simulink model "SHEV_Camaro_PwrLossMdl"  (R2018b)
settings: Solver=ode2  StartTime=0.0  StopTime=simDrv.time_s(end)  FixedStep=t_step  RelTol=1e-3
values from neighbouring files (symbols this model uses):
  A123_ESS =     [PwrLossMdl_A123Battery.mat]
  adj_motEffMap = [0.25 0.31 0.37 0.38 0.4 0.49 0.58 0.64 0.31 0.36 0.39 0.406 ... (72 elements, 8x9)]    [PwrLossMdl_PropSysEffData.mat]
  adjbsfc_map = [1051 1388 1174 1085 895 602 501 388 388 1051 1134 996 ... (81 elements, 9x9)]    [PwrLossMdl_GenSysEffData.mat]
  adjbsfc_spdbpt = [4003 4510 4987 5412 5800 5986 6322 6643 6889]    [PwrLossMdl_GenSysEffData.mat]
  adjbsfc_trqbpt = [10 15 20 25 30 35 40 45 50]    [PwrLossMdl_GenSysEffData.mat]
  C1 = [20000 20000 46318.5184323 46009.1793978 1021.23087801 1108.29786665 9922.48088723 10264.7269718 18293.5148586 29962.1621632 36298.3673472 37544.2700719 ... (41 elements, 1x41)]    [PwrLossMdl_ESS.mat]
  C2 = [20000 20000 46318.5184106 46009.1793608 1021.23035996 1108.29602087 9922.4809203 10264.72697 18293.5148606 29962.1621637 36298.3673482 37544.2700716 ... (41 elements, 1x41)]    [PwrLossMdl_ESS.mat]
  contMotTrq = [250 250 250 250 250 250 225 190 170]    [PwrLossMdl_PropSysEffData.mat]    (also in startPwrLossMdl.m = [180;180;180;180;180;180;180;180;170])
  cs_ll = 0.15    [startPwrLossMdl.m]
  cs_ul = 0.25    [startPwrLossMdl.m]
  E85_LHV = 30000    [startPwrLossMdl.m]
  mot_gbx_rat = 4.2    [startPwrLossMdl.m]
  motSpdVec = [1 500 1000 1500 2000 2500 3000 3500 4000]    [PwrLossMdl_PropSysEffData.mat]
  motTrqVec = [1 25 50 75 100 125 150 175]    [PwrLossMdl_PropSysEffData.mat]
  R0 = [0.5 0.5 0.413858741447 0.181330616185 0.123924684061 0.082623865753 0.114591066521 0.096554690516 0.0949331545326 0.124564294889 0.118490098825 0.107959033825 ... (41 elements, 1x41)]    [PwrLossMdl_ESS.mat]
  R1 = [0.5 0.5 0.513602817558 0.526624804767 0.484906164492 0.489343525408 0.493637128787 0.498122066152 0.500091294983 0.500054252951 0.500314275839 0.500483147312 ... (41 elements, 1x41)]    [PwrLossMdl_ESS.mat]
  R2 = [0.5 0.5 0.513602817535 0.526624804695 0.484906164494 0.489343525401 0.493637128787 0.498122066152 0.500091294984 0.50005425295 0.500314275838 0.500483147311 ... (41 elements, 1x41)]    [PwrLossMdl_ESS.mat]
  rho_fuel_gpL = 783    [startPwrLossMdl.m]
  simDrv = EEC_Single    [startPwrLossMdl.m]
  soc_bpt = [0 0.025 0.05 0.075 0.1 0.125 0.15 0.175 0.2 0.225 0.25 0.275 ... (41 elements, 1x41)]    [PwrLossMdl_ESS.mat]
  t_step = 0.1    [startPwrLossMdl.m]
  tire_rad_m = 0.346    [startPwrLossMdl.m]
  V_fuel_init_gal = 7    [startPwrLossMdl.m]
undefined symbols (not defined in the file or in its folder): DiscIntNeverNeededParam, N_OptResults, OptResults
libraries: simulink x10, custom_func x2, dspstat3 x1
(part 1 of 2)
PauseFcn:
  | runOptSHEV_DP_FwdProp
settings Model: Creator=Aman-Home  LastModifiedBy=Aman-Home

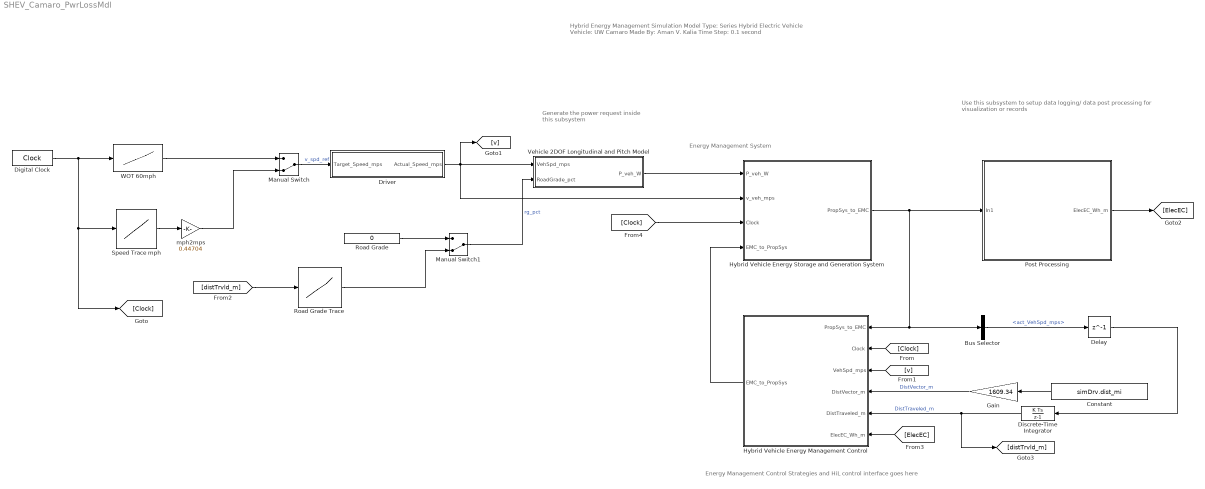
== system SHEV_Camaro_PwrLossMdl ==
  note: Energy Management Control Strategies and HiL control interface goes here
  note: Hybrid Energy Management Simulation Model
      | Type: Series Hybrid Electric Vehicle
      | Vehicle: UW Camaro
      | Made By: Aman V. Kalia
      | Time Step: 0.1 second
  note: Use this subsystem to setup data logging/ data post processing
      | for visualization or records
  note: Generate the power request inside
      | this subsystem
  note: Energy Management System
  Bus Selector : BusSelector  OutputSignals=act_VehSpd_mps
  Constant : Constant  Value=simDrv.dist_mi
  Delay : Delay  DelayLength=1
  Digital Clock : DigitalClock  SampleTime=t_step
  Discrete-Time Integrator : DiscreteIntegrator  SampleTime=t_step  ICPrevOutput=DiscIntNeverNeededParam  ICPrevScaledInput=DiscIntNeverNeededParam
  Driver : Subsystem
  Gain : Gain  Gain=1609.34
  Hybrid Vehicle Energy Management Control : Subsystem
  Hybrid Vehicle Energy Storage and Generation System : Subsystem
  Manual Switch : ManualSwitch  CurrentSetting=0
  Manual Switch1 : ManualSwitch  CurrentSetting=0
  Post Processing : Subsystem
  Road Grade : Constant  Value=0
  Road Grade Trace : Lookup_n-D  NumberOfTableDimensions=1  BreakpointsForDimension1=simDrv.dist_mi(1:end-1) * 1609.34  Table=simDrv.grade_pct(1:end-1)  ExtrapMethod=Clip  UseLastTableValue=on  InternalRulePriority=Speed  RndMeth=Simplest  InputSameDT=on
  Speed Trace mph : Lookup_n-D  NumberOfTableDimensions=1  BreakpointsForDimension1=simDrv.time_s  Table=simDrv.rand_spd_mph  ExtrapMethod=Clip  InternalRulePriority=Speed  RndMeth=Simplest  InputSameDT=on
  Vehicle 2DOF Longitudinal and Pitch Model : Subsystem
  WOT 60mph : Lookup_n-D  NumberOfTableDimensions=1  BreakpointsForDimension1=[0,5,10,simDrv.time_s(end)]  Table=[0,0,60,60] * 0.447  ExtrapMethod=Clip  InternalRulePriority=Speed  RndMeth=Simplest  InputSameDT=on
  mph2mps : Gain  Gain=0.44704
  wires:
  Manual Switch/1 -> Driver/1(Target_Speed_mps)  "v_spd_ref"
  Hybrid Vehicle Energy Management Control/1(EMC_to_PropSys) -> Hybrid Vehicle Energy Storage and Generation System/4(EMC_to_PropSys)
  Hybrid Vehicle Energy Storage and Generation System/1(PropSys_to_EMC) -> Hybrid Vehicle Energy Management Control/1(PropSys_to_EMC), Bus Selector/1, Post Processing/1(In1)
  Vehicle 2DOF Longitudinal and Pitch Model/1(P_veh_W) -> Hybrid Vehicle Energy Storage and Generation System/1(P_veh_W)
  Manual Switch1/1 -> Vehicle 2DOF Longitudinal and Pitch Model/2(RoadGrade_pct)  "rg_pct"
  Digital Clock/1 -> [Clock], Speed Trace mph/1, WOT 60mph/1
  Speed Trace mph/1 -> mph2mps/1
  Road Grade/1 -> Manual Switch1/1
  Road Grade Trace/1 -> Manual Switch1/2
  [Clock] -> Hybrid Vehicle Energy Management Control/2(Clock)
  [v] -> Hybrid Vehicle Energy Management Control/3(VehSpd_mps)
  Constant/1 -> Gain/1
  Bus Selector/1 -> Delay/1  "<act_VehSpd_mps>"
  Discrete-Time Integrator/1 -> [distTrvld_m], Hybrid Vehicle Energy Management Control/5(DistTraveled_m)  "DistTraveled_m"
  Gain/1 -> Hybrid Vehicle Energy Management Control/4(DistVector_m)  "DistVector_m"
  WOT 60mph/1 -> Manual Switch/1
  Post Processing/1(ElecEC_Wh_m) -> [ElecEC]
  [ElecEC] -> Hybrid Vehicle Energy Management Control/6(ElecEC_Wh_m)
  Driver/1(Actual_Speed_mps) -> Hybrid Vehicle Energy Storage and Generation System/2(v_veh_mps), Vehicle 2DOF Longitudinal and Pitch Model/1(VehSpd_mps), [v]
  [Clock] -> Hybrid Vehicle Energy Storage and Generation System/3(Clock)
  mph2mps/1 -> Manual Switch/2
  Delay/1 -> Discrete-Time Integrator/1
  [distTrvld_m] -> Road Grade Trace/1

== system SHEV_Camaro_PwrLossMdl/Driver ==
  Target_Speed_mps : Inport
  Actual_Speed_mps : Outport
  wires:
  Target_Speed_mps/1 -> Actual_Speed_mps/1

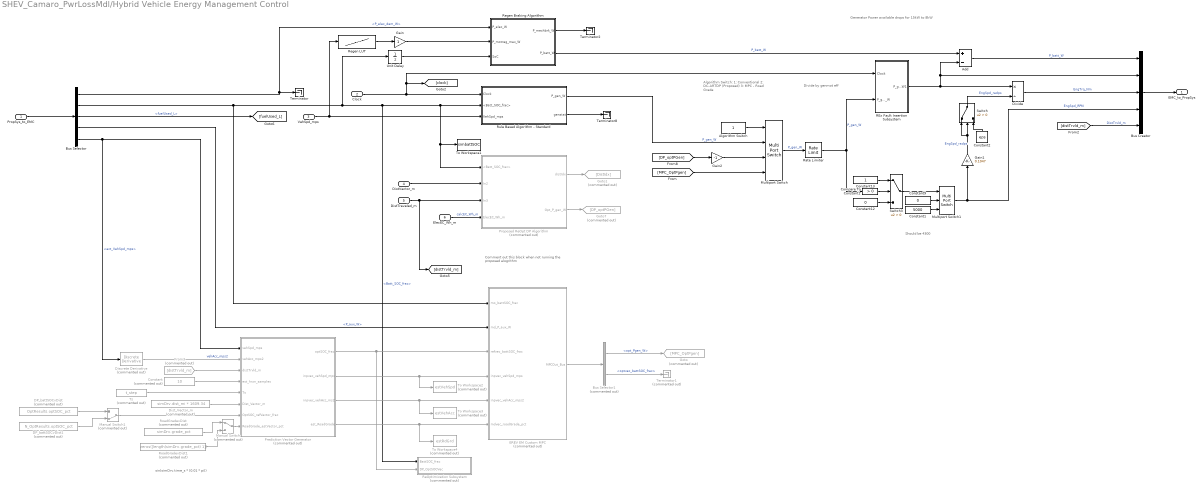
== system SHEV_Camaro_PwrLossMdl/Hybrid Vehicle Energy Management Control ==
  note: Divide by genmot eff
  note: Should be 4300
  note: sin(simDrv.time_s * (0.01 * pi))
  note: Algorithm Switch:
      | 1: Conventional
      | 2: DC-ARTDP (Proposed)
      | 3: MPC - Road Grade
  note: Comment out this block when not
      | running the proposed alogrithm
  note: Generator Power available drops for 15kW to 8kW
  PropSys_to_EMC : Inport
  Clock : Inport  Port=2
  VehSpd_mps : Inport  Port=3
  DistVector_m : Inport  Port=4
  DistTraveled_m : Inport  Port=5
  ElecEC_Wh_m : Inport  Port=6
  Add : Sum  Inputs=+-
  Algorithm Switch : Constant
  Bus Creator : BusCreator  Inputs=5
  Bus Selector : BusSelector  OutputSignals=P_elec_dem_W,Batt_SOC_frac,fuelUsed_L,P_aux_W,act_VehSpd_mps
  Bus Selector1 : BusSelector  Commented=on  OutputSignals=opt_Pgen_W,optvec_battSOC_frac
  Compare To Constant1 : simulink/Logic and Bit Operations/Compare To Constant  relop=>  const=0  OutDataTypeStr=boolean
  Constant : Constant  Commented=on  Value=10
  Constant1 : Constant  Value=5000
  Constant12 : Constant  Value=0
  Constant13 : Constant
  Constant2 : Constant  Value=eps
  Constant9 : Constant  Value=0
  DP_battSOCvDist : Constant  Commented=on  Value=OptResults.optSOC_pct
  DP_battSOCvDist1 : Constant  Commented=on  Value=N_OptResults.optSOC_pct
  Discrete Derivative : simulink/Discrete/Discrete Derivative  Commented=on  gainval=1.0  ICPrevScaledInput=0.0  OutMin=[]  OutMax=[]  OutDataType=fixdt(1, 16)  OutScaling=2^-10  DoSatur=off
  Dist_Vector_m : Constant  Commented=on  Value=simDrv.dist_mi * 1609.34
  Divide : Product  Inputs=*/
  EREV EM Custom MPC : Subsystem  Commented=on  mask{msk_init_Pgen=0, msk_est_hrzn_samples=10, msk_ctl_hrzn_samples=10, msk_t_step=1}
      mask prompts: msk_init_Pgen "Initial generator power [W]:"; msk_est_hrzn_samples "Estimation horizon samples [-]:"; msk_ctl_hrzn_samples "Control horizon samples [-]:"; msk_t_step "Time step [-]:"
      mask DialogControl DescGroupVar Prompt: Custom EREV MPC
      mask DialogControl DescTextVar Prompt: This block implements a custom MPC Energy Management algorithm for the EREV Camaro.
      mask DialogControl ParameterGroupVar Prompt: MPC Parameters
  From3 : From  Commented=on  GotoTag=distTrvld_m
  Gain : Gain
  Gain1 : Gain  Gain=0.1047
  Gain2 : Gain  Gain=-1
  Goto : Goto  Commented=on  GotoTag=MPC_OptPgen
  Goto1 : Goto  Commented=on  GotoTag=DistIdx
  Goto7 : Goto  Commented=on  GotoTag=DP_optPGen
  Manual Switch : ManualSwitch  Commented=on
  Manual Switch1 : ManualSwitch  Commented=on  CurrentSetting=0
  Multiport Switch : MultiPortSwitch
  Multiport Switch1 : MultiPortSwitch  DataPortOrder=Zero-based contiguous  Inputs=2  zeroidx=on
  Prediction Vector Generator : Subsystem  Commented=on
  Proposed ReOpt DP Algorithm : Subsystem  Commented=on
  REx Fault Insertion Subsystem : Subsystem  mask{FaultTypes=No Fault, t_shutfault=6000}
      mask prompts: FaultTypes "Select Fault Type:"; t_shutfault "Enter the time marker [s]:"
      mask init:
      | switch FaultTypes
      |     case 'No Fault'
      |         FaultDec = 0;
      |         %set_param('SHEV_Camaro_PwrLossMdl/Hybrid Vehicle Energy Management Control/Fault Insertion Subsystem','choice','0')
      |     case 'Deration Fault'
      |         FaultDec = 1;
      |         %set_param('SHEV_Camaro_PwrLossMdl/Hybrid Vehicle Energy Management Control/REx Fault Insertion Subsystem','choice','1')
      |     case 'Shut Down Fault'
      |         FaultDec = 2;
      |         %set_param('SHEV_Camaro_PwrLossMdl/Hybrid Vehicle Energy Management Control/Fault Insertion Subsystem','choice','2')
      | end
      mask TypeOptions FaultTypes: No Fault | Deration Fault | Shut Down Fault
      mask Callback FaultTypes:
      | % Get the mask parameter values. This is a cell
      | %   array of character vectors.
      | maskStr = get_param(gcb,'FaultTypes');
      | 
      | % The pop-up menu is the first mask parameter.
      | %   Check the value selected in the pop-up
      | if strcmp(maskStr(1),'S'),
      | 
      |     % Set the visibility of both parameters on when
      |     %   User-defined is selected in the pop-up.
      | 
      |     set_param(gcb,'MaskVisibilities',{'on';'on'}),
      | 
      | else
      | 
      |     % Turn off the visibility of the Value field
      |     %   when User-defined is not selected.
      | 
      |     set_param(gcb,'MaskVisibilities',{'on';'off'}),
      | 
      |     % Set the character vector in the Values field equal to the
      |     % character vector selected in the Gain pop-up menu.
      | 
      |     %maskStr{2}=maskStr{1};
      |     %set_param(gcb,'t_shutfault',inf);
      | end
      mask DialogControl DescGroupVar Prompt: Fault Insertion Block
      mask DialogControl DescTextVar Prompt: Select "Insert Fault" to enable fault insertion. Deselect to turn it off.
      mask DialogControl DescVar Prompt: Select the fault level [0,1,2] using the dial below. [0: No Fault, 1: Deration Fault, 2: Shut Off]
  Rate Limiter : RateLimiter  RisingSlewLimit=250  FallingSlewLimit=-4500  SampleTimeMode=inherited
  ReOptimization Subsystem : Subsystem  Commented=on
  Regen Braking Algorithm : Stateflow chart  TreatAsAtomicUnit=on
  Regen LUT : Lookup_n-D  NumberOfTableDimensions=1  BreakpointsForDimension1=[0 2.6 5.2 7.8 10.4 13 15.6 18.2 20.8 23.4 26 28.6 31.2 33.8 38]  Table=[0 0 -1250 -3000 -5500 -8000 -10250 -12500 -13750 -14000 -14500 -15000 -15000 -15000 -15000]  InternalRulePriority=Speed  RndMeth=Simplest  InputSameDT=on
  RoadGradevDist : Constant  Commented=on  Value=simDrv.grade_pct
  RoadGradevDist1 : Constant  Commented=on  Value=zeros([length(simDrv.grade_pct) 1])
  Rule Based Algorithm - Standard : Subsystem
  Switch : Switch  Criteria=u2 > Threshold
  Switch3 : Switch  Criteria=u2 > Threshold
  Terminator : Terminator
  Terminator1 : Terminator  Commented=on
  Terminator2 : Terminator
  Terminator8 : Terminator
  To Workspace1 : ToWorkspace  VariableName=simbattSOC  SaveFormat=Timeseries  SampleTime=1
  To Workspace2 : ToWorkspace  Commented=on  VariableName=estVehSpd  SaveFormat=Structure With Time  SampleTime=-1
      settings: Save2DSignal=2-D array (concatenate along first dimension)
  To Workspace3 : ToWorkspace  Commented=on  VariableName=estVehAcc  SaveFormat=Structure With Time  SampleTime=-1
      settings: Save2DSignal=2-D array (concatenate along first dimension)
  To Workspace4 : ToWorkspace  Commented=on  VariableName=estRdGrd  SaveFormat=Structure With Time  SampleTime=-1
      settings: Save2DSignal=2-D array (concatenate along first dimension)
  Ts : Constant  Commented=on  Value=t_step
  Unit Delay : UnitDelay  SampleTime=-1
  EMC_to_PropSys : Outport
  wires:
  Bus Creator/1 -> EMC_to_PropSys/1
  Add/1 -> Bus Creator/1  "P_batt_W"
  Divide/1 -> Bus Creator/3  "EngTrq_Nm"
  Multiport Switch1/1 -> Gain1/1, Bus Creator/4  "EngSpd_RPM"
  PropSys_to_EMC/1 -> Bus Selector/1
  Bus Selector/1 -> Terminator/1, Regen Braking Algorithm/1(P_elec_W)  "<P_elec_dem_W>"
  Regen LUT/1 -> Gain/1
  Regen Braking Algorithm/1(P_mechbrk_W) -> Terminator2/1
  Gain/1 -> Regen Braking Algorithm/2(P_motreg_max_W)
  Constant9/1 -> Multiport Switch1/2
  Constant1/1 -> Multiport Switch1/3
  Switch/1 -> Divide/2  "EngSpd_radps"
  Gain1/1 -> Switch/1, Switch/2  "EngSpd_radps"
  Constant2/1 -> Switch/3
  Regen Braking Algorithm/2(P_batt_W) -> Add/1  "P_batt_W"
  Clock/1 -> Rule Based Algorithm - Standard/1(Clock), REx Fault Insertion Subsystem/1(Clock), [clock]
  Bus Selector/2 -> EREV EM Custom MPC/1(mo_battSOC_frac), ReOptimization Subsystem/1(BattSOC_frac), Rule Based Algorithm - Standard/2(<Batt_SOC_frac>), Proposed ReOpt DP Algorithm/1(<Batt_SOC_frac>), To Workspace1/1, Unit Delay/1  "<Batt_SOC_frac>"
  VehSpd_mps/1 -> Rule Based Algorithm - Standard/3(VehSpd_mps), Regen LUT/1
  Switch3/1 -> Multiport Switch1/1
  DistTraveled_m/1 -> Proposed ReOpt DP Algorithm/3(In3), [distTrvld_m]
  Bus Selector/3 -> [fuelUsed_L]  "<fuelUsed_L>"
  [DP_optPGen] -> Gain2/1
  Gain2/1 -> Multiport Switch/3
  Rule Based Algorithm - Standard/1(P_gen_W) -> Multiport Switch/2  "P_gen_W"
  Algorithm Switch/1 -> Multiport Switch/1
  Rule Based Algorithm - Standard/2(genstat) -> Terminator8/1
  Compare To Constant1/1 -> Switch3/2
  Constant12/1 -> Switch3/3
  Constant13/1 -> Switch3/1
  [distTrvld_m] -> Bus Creator/5  "DistTrvld_m"
  Unit Delay/1 -> Regen Braking Algorithm/3(SoC)
  REx Fault Insertion Subsystem/1(P_gen_W1) -> Add/2, Bus Creator/2, Divide/1
  Rate Limiter/1 -> Compare To Constant1/1, REx Fault Insertion Subsystem/2(P_gen_W)  "P_gen_W"
  DistVector_m/1 -> Proposed ReOpt DP Algorithm/2(In2)
  ElecEC_Wh_m/1 -> Proposed ReOpt DP Algorithm/4(ElecEC_Wh_m)  "calcEC_Wh_m"
  Proposed ReOpt DP Algorithm/1(distIdx) -> Goto1/1
  Proposed ReOpt DP Algorithm/2(Opt_P_gen_W) -> Goto7/1
  [MPC_OptPgen] -> Multiport Switch/4
  EREV EM Custom MPC/1(MPCOut_Bus) -> Bus Selector1/1
  Bus Selector1/1 -> Goto/1  "<opt_Pgen_W>"
  Bus Selector1/2 -> Terminator1/1  "<optvec_battSOC_frac>"
  Bus Selector/4 -> EREV EM Custom MPC/2(md_P_aux_W)  "<P_aux_W>"
  Prediction Vector Generator/1(optSOC_frac) -> ReOptimization Subsystem/2(DP_OptSOCVec), EREV EM Custom MPC/3(refvec_battSOC_frac)
  Prediction Vector Generator/2(inpvec_vehSpd_mps) -> To Workspace2/1, EREV EM Custom MPC/4(inpvec_vehSpd_mps)
  Prediction Vector Generator/3(inpvec_vehAcc_ms2) -> To Workspace3/1, EREV EM Custom MPC/5(inpvec_vehAcc_mps2)
  Prediction Vector Generator/4(est_RoadGrade) -> To Workspace4/1, EREV EM Custom MPC/6(mdvec_roadGrade_pct)
  From3/1 -> Prediction Vector Generator/3(distTrvld_m)
  Constant/1 -> Prediction Vector Generator/4(est_hrzn_samples)
  RoadGradevDist/1 -> Manual Switch/1
  Manual Switch1/1 -> Prediction Vector Generator/7(OptSOC_refVector_frac)
  Dist_Vector_m/1 -> Prediction Vector Generator/6(Dist_Vector_m)
  Ts/1 -> Prediction Vector Generator/5(Ts)
  Bus Selector/5 -> Discrete Derivative/1, Prediction Vector Generator/1(vehSpd_mps)  "<act_VehSpd_mps>"
  Discrete Derivative/1 -> Prediction Vector Generator/2(vehAcc_mps2)  "vehAcc_mps2"
  Manual Switch/1 -> Prediction Vector Generator/8(RoadGrade_estVector_pct)
  RoadGradevDist1/1 -> Manual Switch/2
  DP_battSOCvDist/1 -> Manual Switch1/1
  DP_battSOCvDist1/1 -> Manual Switch1/2
  Multiport Switch/1 -> Rate Limiter/1  "P_gen_W"

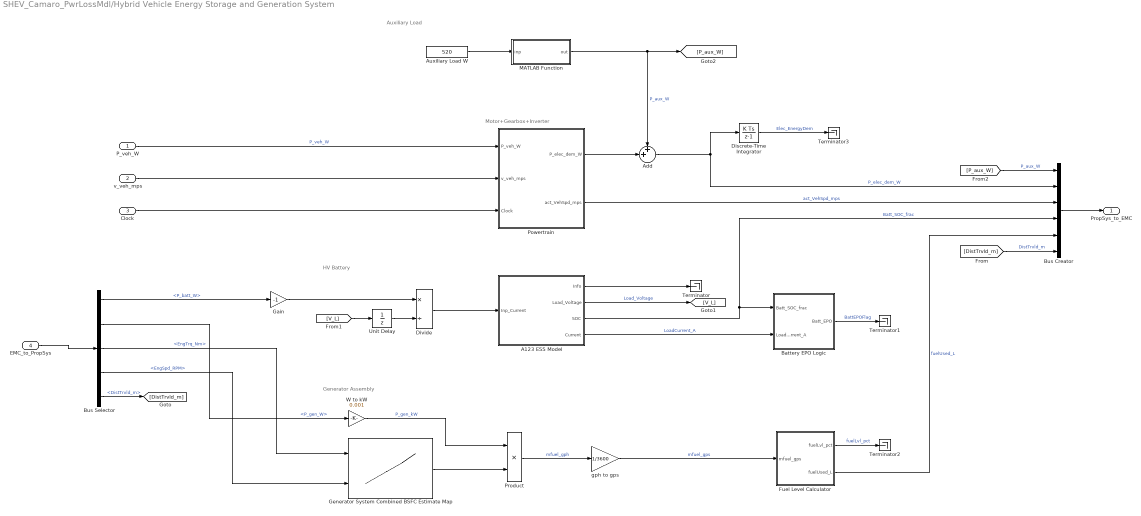
== system SHEV_Camaro_PwrLossMdl/Hybrid Vehicle Energy Storage and Generation System ==
  note: HV Battery
  note: Generator Assembly
  note: Auxiliary Load
  note: Motor+Gearbox+Inverter
  P_veh_W : Inport
  v_veh_mps : Inport  Port=2
  Clock : Inport  Port=3
  EMC_to_PropSys : Inport  Port=4
  A123 ESS Model : Subsystem  AncestorBlock=lib_ESS/A123 ESS Model  mask{Q_max_cell=A123_ESS.Q_cell_max_Ah, Np=A123_ESS.Np, Ns=A123_ESS.Ns, Nmod=A123_ESS.Nmod, soc_init=A123_ESS.Init_soc, soc_bpt=soc_bpt, R0=R0, R1=R1, C1=C1, R2=R2, C2=C2, t_step=t_step}
      mask prompts: Q_max_cell "Max cell capacity [Ah]:"; Np "Number of cells in parallel []:"; Ns "Numer of cells in series []:"; Nmod "Number of modules []:"; soc_init "Initial SoC/100 []:"; soc_bpt "SoC break points []:"; R0 "Internal resistance vector []:"; R1 "RC1 resistance vector []:"; C1 "RC1 capacitance vector []:"; R2 "RC2 resistance vector []:"; C2 "RC2 capacitance vector []:"; t_step "Simulation time step:"
      mask DialogControl DescGroupVar Prompt: Parameter Settings
      mask DialogControl DescTextVar Prompt: This model emulates an A123 ESS used by UW EcoCAR Team.
      mask DialogControl BatParamGroupVar Prompt: Battery Parameters
      mask DialogControl EstParamGroupVar Prompt: Estimated RC Parameters
      mask DialogControl MiscSettGroupVar Prompt: Miscellaneous Settings
  Add : Sum  Inputs=++|
  Auxiliary Load W : Constant  Value=520
  Battery EPO Logic : Subsystem
  Bus Creator : BusCreator  Inputs=6
  Bus Selector : BusSelector  OutputSignals=P_batt_W,P_gen_W,EngTrq_Nm,EngSpd_RPM,DistTrvld_m
  Discrete-Time Integrator : DiscreteIntegrator  SampleTime=t_step  ICPrevOutput=DiscIntNeverNeededParam  ICPrevScaledInput=DiscIntNeverNeededParam
  Divide : Product  Inputs=*/
  Fuel Level Calculator : Subsystem
  Gain : Gain  Gain=-1
  Generator System Combined BSFC Estimate Map : Lookup_n-D  BreakpointsForDimension1=adjbsfc_trqbpt  BreakpointsForDimension2=adjbsfc_spdbpt  Table=adjbsfc_map  InternalRulePriority=Speed  RndMeth=Simplest  InputSameDT=on
  MATLAB Function : MATLAB Function  TreatAsAtomicUnit=on
  Powertrain : Subsystem
  Product : Product
  Terminator{,1..3} (4 alike) : Terminator
  Unit Delay : UnitDelay  InitialCondition=A123_ESS.Ns * A123_ESS.Nmod * 3.4  SampleTime=-1
  W to kW : Gain  Gain=0.001
  gph to gps : Gain  Gain=1/3600
  PropSys_to_EMC : Outport
  wires:
  P_veh_W/1 -> Powertrain/1(P_veh_W)  "P_veh_W"
  v_veh_mps/1 -> Powertrain/2(v_veh_mps)
  Auxiliary Load W/1 -> MATLAB Function/1(inp)
  Powertrain/1(P_elec_dem_W) -> Add/2
  MATLAB Function/1(out) -> Add/1, [P_aux_W]  "P_aux_W"
  Add/1 -> Bus Creator/2, Discrete-Time Integrator/1  "P_elec_dem_W"
  Divide/1 -> A123 ESS Model/1(Inp_Current)
  A123 ESS Model/2(Load_Voltage) -> [V_L]  "Load_Voltage"
  [V_L] -> Unit Delay/1
  A123 ESS Model/1(Info) -> Terminator/1
  A123 ESS Model/3(SOC) -> Bus Creator/4, Battery EPO Logic/1(Batt_SOC_frac)  "Batt_SOC_frac"
  Bus Selector/3 -> Generator System Combined BSFC Estimate Map/1  "<EngTrq_Nm>"
  Bus Selector/4 -> Generator System Combined BSFC Estimate Map/2  "<EngSpd_RPM>"
  EMC_to_PropSys/1 -> Bus Selector/1
  Bus Selector/1 -> Gain/1  "<P_batt_W>"
  Bus Selector/2 -> W to kW/1  "<P_gen_W>"
  Generator System Combined BSFC Estimate Map/1 -> Product/2
  W to kW/1 -> Product/1  "P_gen_kW"
  Product/1 -> gph to gps/1  "mfuel_gph"
  Bus Creator/1 -> PropSys_to_EMC/1
  Unit Delay/1 -> Divide/2
  Gain/1 -> Divide/1
  A123 ESS Model/4(Current) -> Battery EPO Logic/2(LoadCurrent_A)  "LoadCurrent_A"
  Battery EPO Logic/1(Batt_EPO) -> Terminator1/1  "BattEPOFlag"
  gph to gps/1 -> Fuel Level Calculator/1(mfuel_gps)  "mfuel_gps"
  Fuel Level Calculator/1(fuelLvl_pct) -> Terminator2/1  "fuelLvl_pct"
  Discrete-Time Integrator/1 -> Terminator3/1  "Elec_EnergyDem"
  Fuel Level Calculator/2(fuelUsed_L) -> Bus Creator/5  "fuelUsed_L"
  Bus Selector/5 -> [DistTrvld_m]  "<DistTrvld_m>"
  [DistTrvld_m] -> Bus Creator/6  "DistTrvld_m"
  Clock/1 -> Powertrain/3(Clock)
  Powertrain/2(act_VehSpd_mps) -> Bus Creator/3  "act_VehSpd_mps"
  [P_aux_W] -> Bus Creator/1  "P_aux_W"

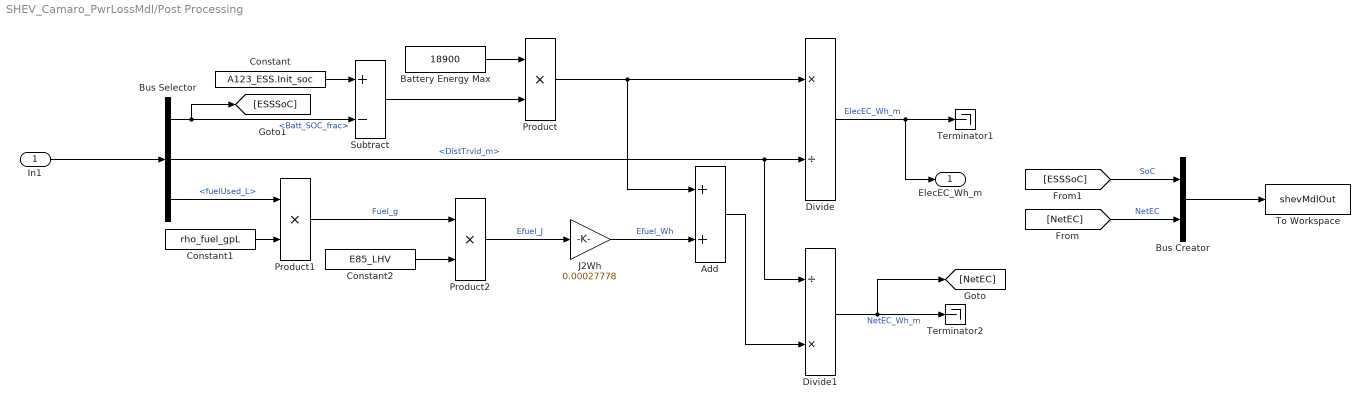
== system SHEV_Camaro_PwrLossMdl/Post Processing ==
  In1 : Inport
  Add : Sum
  Battery Energy Max : Constant  Value=18900
  Bus Creator : BusCreator  Inputs=2
  Bus Selector : BusSelector  OutputSignals=Batt_SOC_frac,DistTrvld_m,fuelUsed_L
  Constant : Constant  Value=A123_ESS.Init_soc
  Constant1 : Constant  Value=rho_fuel_gpL
  Constant2 : Constant  Value=E85_LHV
  Divide : Product  Inputs=*/
  Divide1 : Product  Inputs=/*
  J2Wh : Gain  Gain=0.00027778
  Product : Product
  Product1 : Product
  Product2 : Product
  Subtract : Sum  Inputs=+-
  Terminator1 : Terminator
  Terminator2 : Terminator
  To Workspace : ToWorkspace  VariableName=shevMdlOut  SaveFormat=Timeseries  SampleTime=-1
  ElecEC_Wh_m : Outport
  wires:
  In1/1 -> Bus Selector/1
  Bus Selector/1 -> [ESSSoC], Subtract/2  "<Batt_SOC_frac>"
  Constant/1 -> Subtract/1
  Subtract/1 -> Product/2
  Battery Energy Max/1 -> Product/1
  Product/1 -> Add/1, Divide/1
  Bus Selector/2 -> Divide1/1, Divide/2  "<DistTrvld_m>"
  Bus Selector/3 -> Product1/1  "<fuelUsed_L>"
  Divide/1 -> ElecEC_Wh_m/1, Terminator1/1  "ElecEC_Wh_m"
  Constant1/1 -> Product1/2
  Product1/1 -> Product2/1  "Fuel_g"
  Constant2/1 -> Product2/2
  Product2/1 -> J2Wh/1  "Efuel_J"
  J2Wh/1 -> Add/2  "Efuel_Wh"
  Add/1 -> Divide1/2
  Divide1/1 -> [NetEC], Terminator2/1  "NetEC_Wh_m"
  Bus Creator/1 -> To Workspace/1
  [NetEC] -> Bus Creator/2  "NetEC"
  [ESSSoC] -> Bus Creator/1  "SoC"

== system SHEV_Camaro_PwrLossMdl/Vehicle 2DOF Longitudinal and Pitch Model ==
  VehSpd_mps : Inport
  RoadGrade_pct : Inport  Port=2
  Simulation Time Step : Constant  Value=t_step
  Terminator{,1..6} (7 alike) : Terminator
  Vehicle Dynamics Model 2 DOF (Longitudinal and Pitch) : MATLAB Function  TreatAsAtomicUnit=on
  P_veh_W : Outport
  wires:
  VehSpd_mps/1 -> Vehicle Dynamics Model 2 DOF (Longitudinal and Pitch)/1(v_spd)
  Vehicle Dynamics Model 2 DOF (Longitudinal and Pitch)/1(P_veh) -> P_veh_W/1  "P_veh"
  RoadGrade_pct/1 -> Vehicle Dynamics Model 2 DOF (Longitudinal and Pitch)/2(rg_pct)
  Simulation Time Step/1 -> Vehicle Dynamics Model 2 DOF (Longitudinal and Pitch)/3(dt)
  Vehicle Dynamics Model 2 DOF (Longitudinal and Pitch)/2(Trq_dem) -> Terminator/1  "MotTrqDem_Nm"
  Vehicle Dynamics Model 2 DOF (Longitudinal and Pitch)/3(acc_veh) -> Terminator1/1  "VehAcc_ms2"
  Vehicle Dynamics Model 2 DOF (Longitudinal and Pitch)/4(KE_veh) -> Terminator2/1  "PowKE_Vehicle"
  Vehicle Dynamics Model 2 DOF (Longitudinal and Pitch)/5(Pwr_RR) -> Terminator3/1  "Pwr_RR"
  Vehicle Dynamics Model 2 DOF (Longitudinal and Pitch)/6(Pwr_Load) -> Terminator4/1  "Pwr_Load"
  Vehicle Dynamics Model 2 DOF (Longitudinal and Pitch)/7(dist_m) -> Terminator5/1  "Distance_m"
  Vehicle Dynamics Model 2 DOF (Longitudinal and Pitch)/8(elev_m) -> Terminator6/1  "Elevation_m"

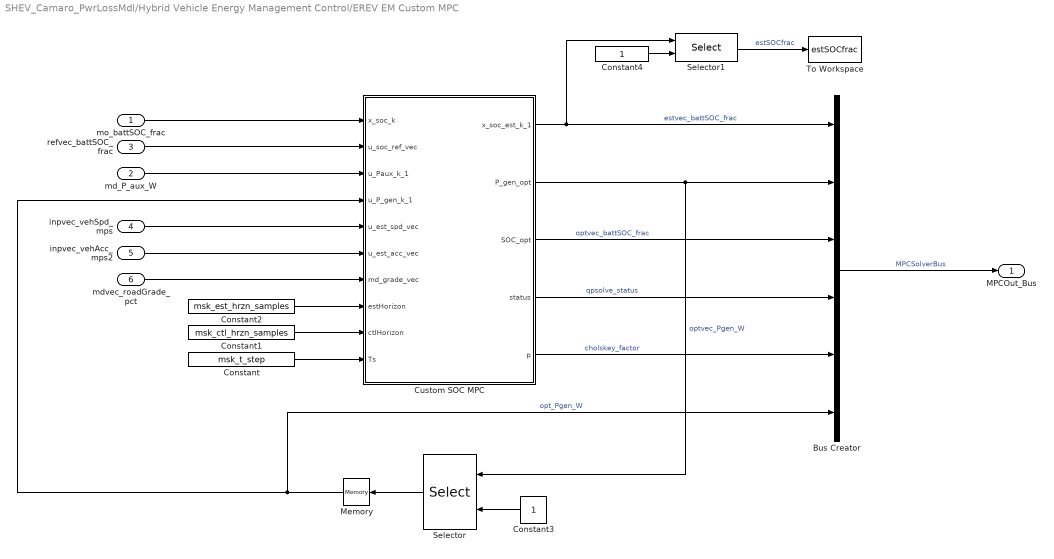
== system SHEV_Camaro_PwrLossMdl/Hybrid Vehicle Energy Management Control/EREV EM Custom MPC ==
  mo_battSOC_frac : Inport
  md_P_aux_W : Inport  Port=2
  refvec_battSOC_frac : Inport  Port=3
  inpvec_vehSpd_mps : Inport  Port=4
  inpvec_vehAcc_mps2 : Inport  Port=5
  mdvec_roadGrade_pct : Inport  Port=6
  Bus Creator : BusCreator  Inputs=6
  Constant : Constant  Value=msk_t_step
  Constant1 : Constant  Value=msk_ctl_hrzn_samples
  Constant2 : Constant  Value=msk_est_hrzn_samples
  Constant3 : Constant
  Constant4 : Constant
  Custom SOC MPC : MATLAB Function  TreatAsAtomicUnit=on
  Memory : Memory  InitialCondition=msk_init_Pgen  InheritSampleTime=on  LinearizeAsDelay=on
  Selector : Selector  InputPortWidth=30  IndexOptions=Index vector (port)  Indices=[1 3]  OutputSizes=1
  Selector1 : Selector  InputPortWidth=30  IndexOptions=Index vector (port)  Indices=[1 3]  OutputSizes=1
  To Workspace : ToWorkspace  VariableName=estSOCfrac  SaveFormat=Timeseries  SampleTime=-1
  MPCOut_Bus : Outport
  wires:
  Constant/1 -> Custom SOC MPC/10(Ts)
  Custom SOC MPC/2(P_gen_opt) -> Selector/1, Bus Creator/2  "optvec_Pgen_W"
  Custom SOC MPC/3(SOC_opt) -> Bus Creator/3  "optvec_battSOC_frac"
  md_P_aux_W/1 -> Custom SOC MPC/3(u_Paux_k_1)
  mdvec_roadGrade_pct/1 -> Custom SOC MPC/7(md_grade_vec)
  Constant2/1 -> Custom SOC MPC/8(estHorizon)
  mo_battSOC_frac/1 -> Custom SOC MPC/1(x_soc_k)
  Custom SOC MPC/1(x_soc_est_k_1) -> Selector1/1, Bus Creator/1  "estvec_battSOC_frac"
  refvec_battSOC_frac/1 -> Custom SOC MPC/2(u_soc_ref_vec)
  Custom SOC MPC/5(p) -> Bus Creator/5  "cholskey_factor"
  inpvec_vehAcc_mps2/1 -> Custom SOC MPC/6(u_est_acc_vec)
  inpvec_vehSpd_mps/1 -> Custom SOC MPC/5(u_est_spd_vec)
  Constant1/1 -> Custom SOC MPC/9(ctlHorizon)
  Custom SOC MPC/4(status) -> Bus Creator/4  "qpsolve_status"
  Bus Creator/1 -> MPCOut_Bus/1  "MPCSolverBus"
  Constant3/1 -> Selector/2
  Selector/1 -> Memory/1
  Memory/1 -> Bus Creator/6, Custom SOC MPC/4(u_P_gen_k_1)  "opt_Pgen_W"
  Constant4/1 -> Selector1/2
  Selector1/1 -> To Workspace/1  "estSOCfrac"

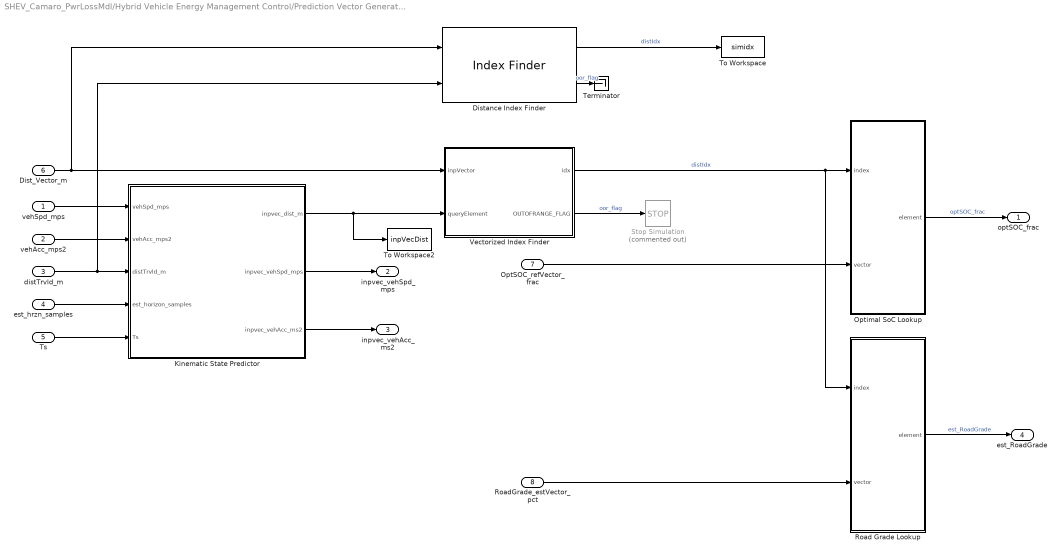
== system SHEV_Camaro_PwrLossMdl/Hybrid Vehicle Energy Management Control/Prediction Vector Generator ==
  vehSpd_mps : Inport
  vehAcc_mps2 : Inport  Port=2
  distTrvld_m : Inport  Port=3
  est_hrzn_samples : Inport  Port=4
  Ts : Inport  Port=5
  Dist_Vector_m : Inport  Port=6
  OptSOC_refVector_frac : Inport  Port=7
  RoadGrade_estVector_pct : Inport  Port=8
  Distance Index Finder : custom_func/Index Finder  SystemSampleTime=-1
  Kinematic State Predictor : MATLAB Function  TreatAsAtomicUnit=on
  Optimal SoC Lookup : MATLAB Function  TreatAsAtomicUnit=on
  Road Grade Lookup : MATLAB Function  TreatAsAtomicUnit=on
  Stop Simulation : Stop  Commented=on
  Terminator : Terminator
  To Workspace : ToWorkspace  VariableName=simidx  SaveFormat=Timeseries  SampleTime=1
      settings: Save2DSignal=2-D array (concatenate along first dimension)
  To Workspace2 : ToWorkspace  VariableName=inpVecDist  SaveFormat=Structure With Time  SampleTime=-1
      settings: Save2DSignal=2-D array (concatenate along first dimension)
  Vectorized Index Finder : MATLAB Function  TreatAsAtomicUnit=on
  optSOC_frac : Outport
  inpvec_vehSpd_mps : Outport  Port=2
  inpvec_vehAcc_ms2 : Outport  Port=3
  est_RoadGrade : Outport  Port=4
  wires:
  Road Grade Lookup/1(element) -> est_RoadGrade/1  "est_RoadGrade"
  OptSOC_refVector_frac/1 -> Optimal SoC Lookup/2(vector)
  Kinematic State Predictor/1(inpvec_dist_m) -> To Workspace2/1, Vectorized Index Finder/2(queryElement)
  Vectorized Index Finder/2(OUTOFRANGE_FLAG) -> Stop Simulation/1  "oor_flag"
  Vectorized Index Finder/1(idx) -> Road Grade Lookup/1(index), Optimal SoC Lookup/1(index)  "distIdx"
  RoadGrade_estVector_pct/1 -> Road Grade Lookup/2(vector)
  Optimal SoC Lookup/1(element) -> optSOC_frac/1  "optSOC_frac"
  Dist_Vector_m/1 -> Distance Index Finder/1, Vectorized Index Finder/1(inpVector)
  Kinematic State Predictor/2(inpvec_vehSpd_mps) -> inpvec_vehSpd_mps/1
  Kinematic State Predictor/3(inpvec_vehAcc_ms2) -> inpvec_vehAcc_ms2/1
  vehSpd_mps/1 -> Kinematic State Predictor/1(vehSpd_mps)
  distTrvld_m/1 -> Distance Index Finder/2, Kinematic State Predictor/3(distTrvld_m)
  est_hrzn_samples/1 -> Kinematic State Predictor/4(est_horizon_samples)
  Ts/1 -> Kinematic State Predictor/5(Ts)
  vehAcc_mps2/1 -> Kinematic State Predictor/2(vehAcc_mps2)
  Distance Index Finder/2 -> Terminator/1  "oor_flag"
  Distance Index Finder/1 -> To Workspace/1  "distIdx"

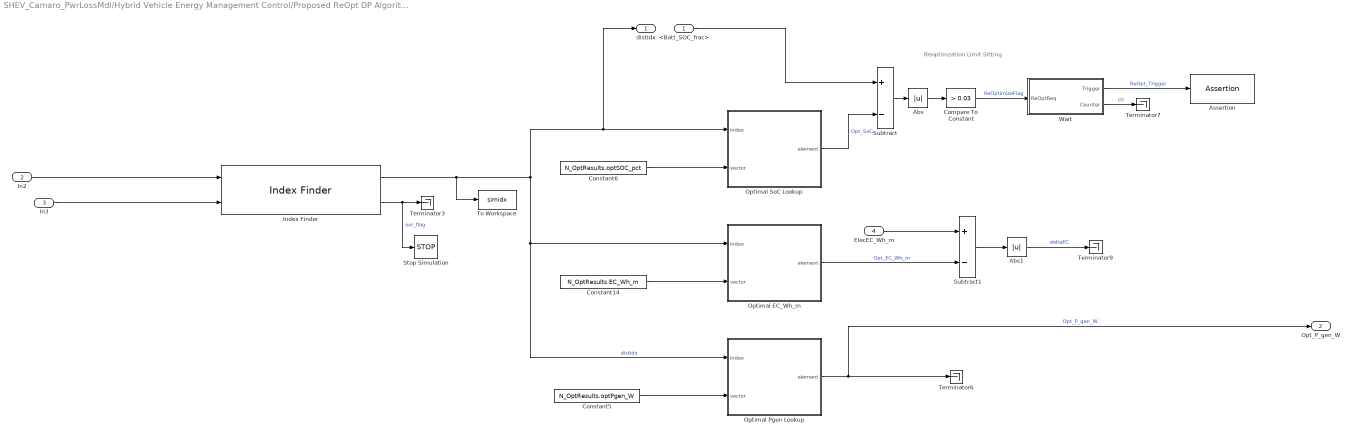
== system SHEV_Camaro_PwrLossMdl/Hybrid Vehicle Energy Management Control/Proposed ReOpt DP Algorithm ==
  note: Reoptimzation Limit Sitting
  <Batt_SOC_frac> : Inport
  In2 : Inport  Port=2
  In3 : Inport  Port=3
  ElecEC_Wh_m : Inport  Port=4
  Abs : Abs
  Abs1 : Abs
  Assertion : Assertion  AssertionFailFcn=set_param(bdroot,'SimulationCommand','pause');  StopWhenAssertionFail=off
  Compare To Constant : simulink/Logic and Bit Operations/Compare To Constant  relop=>  const=0.03  OutDataTypeStr=boolean
  Constant14 : Constant  Value=N_OptResults.EC_Wh_m
  Constant5 : Constant  Value=N_OptResults.optPgen_W
  Constant6 : Constant  Value=N_OptResults.optSOC_pct
  Index Finder : custom_func/Index Finder  SystemSampleTime=-1
  Optimal EC_Wh_m : MATLAB Function  TreatAsAtomicUnit=on
  Optimal Pgen Lookup : MATLAB Function  TreatAsAtomicUnit=on
  Optimal SoC Lookup : MATLAB Function  TreatAsAtomicUnit=on
  Stop Simulation : Stop
  Subtract : Sum  Inputs=+-
  Subtract1 : Sum  Inputs=+-
  Terminator{3,6..7,9} (4 alike) : Terminator
  To Workspace : ToWorkspace  VariableName=simidx  SaveFormat=Timeseries  SampleTime=1
      settings: Save2DSignal=2-D array (concatenate along first dimension)
  Wait : Stateflow chart  TreatAsAtomicUnit=on
  distIdx : Outport
  Opt_P_gen_W : Outport  Port=2
  wires:
  In3/1 -> Index Finder/2
  <Batt_SOC_frac>/1 -> Subtract/1
  Abs1/1 -> Terminator9/1  "deltaEC"
  In2/1 -> Index Finder/1
  Subtract/1 -> Abs/1
  Constant6/1 -> Optimal SoC Lookup/2(vector)
  Compare To Constant/1 -> Wait/1(ReOptReq)  "ReOptimizeFlag"
  Abs/1 -> Compare To Constant/1
  Index Finder/1 -> To Workspace/1, distIdx/1, Optimal SoC Lookup/1(index), Optimal EC_Wh_m/1(index), Optimal Pgen Lookup/1(index)  "distIdx"
  ElecEC_Wh_m/1 -> Subtract1/1
  Optimal SoC Lookup/1(element) -> Subtract/2  "Opt_SoC"
  Optimal EC_Wh_m/1(element) -> Subtract1/2  "Opt_EC_Wh_m"
  Subtract1/1 -> Abs1/1
  Wait/2(Counter) -> Terminator7/1  "ctr"
  Optimal Pgen Lookup/1(element) -> Opt_P_gen_W/1, Terminator6/1  "Opt_P_gen_W"
  Index Finder/2 -> Terminator3/1, Stop Simulation/1  "oor_flag"
  Constant5/1 -> Optimal Pgen Lookup/2(vector)
  Wait/1(Trigger) -> Assertion/1  "ReOpt_Trigger"
  Constant14/1 -> Optimal EC_Wh_m/2(vector)

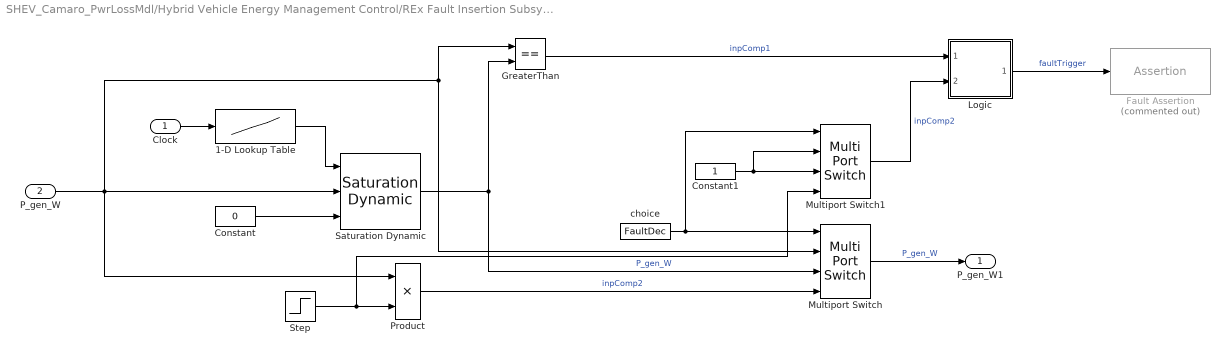
== system SHEV_Camaro_PwrLossMdl/Hybrid Vehicle Energy Management Control/REx Fault Insertion Subsystem ==
  Clock : Inport
  P_gen_W : Inport  Port=2
  1-D Lookup Table : Lookup_n-D  NumberOfTableDimensions=1  BreakpointsForDimension1=[0,100,101,simDrv.time_s(end)]  Table=[15000,15000,15000,15000]  InternalRulePriority=Speed  RndMeth=Simplest  InputSameDT=on
  Constant : Constant  Value=0
  Constant1 : Constant
  Fault Assertion : Assertion  Commented=on  AssertionFailFcn=|  StopWhenAssertionFail=off
      | set_param(bdroot,'SimulationCommand','pause');
      | disp('## Paused due to REx fault insertion')
  GreaterThan : RelationalOperator  Operator===  OutDataTypeStr=boolean  RndMeth=Simplest
  Logic : Stateflow chart  TreatAsAtomicUnit=on
  Multiport Switch : MultiPortSwitch  DataPortOrder=Zero-based contiguous  zeroidx=on
  Multiport Switch1 : MultiPortSwitch  DataPortOrder=Zero-based contiguous  zeroidx=on
  Product : Product
  Saturation Dynamic : simulink/Discontinuities/Saturation Dynamic  OutMin=[]  OutMax=[]  OutDataTypeStr=Inherit: Same as second input  OutDataType=fixdt(1, 16)  OutScaling=2^-10  DoSatur=off
  Step : Step  Time=t_shutfault  Before=1  After=0  SampleTime=t_step
  choice : Constant  Value=FaultDec
  P_gen_W1 : Outport
  wires:
  Multiport Switch/1 -> P_gen_W1/1  "P_gen_W"
  Constant/1 -> Saturation Dynamic/3
  Clock/1 -> 1-D Lookup Table/1
  P_gen_W/1 -> Product/1, Saturation Dynamic/2, Multiport Switch/2, GreaterThan/1
  1-D Lookup Table/1 -> Saturation Dynamic/1
  Saturation Dynamic/1 -> GreaterThan/2, Multiport Switch/3  "P_gen_W"
  choice/1 -> Multiport Switch1/1, Multiport Switch/1
  GreaterThan/1 -> Logic/1(input1)  "inpComp1"
  Logic/1(trigger) -> Fault Assertion/1  "faultTrigger"
  Product/1 -> Multiport Switch/4  "inpComp2"
  Step/1 -> Multiport Switch1/4, Product/2
  Multiport Switch1/1 -> Logic/2(input2)  "inpComp2"
  Constant1/1 -> Multiport Switch1/2, Multiport Switch1/3

== system SHEV_Camaro_PwrLossMdl/Hybrid Vehicle Energy Management Control/ReOptimization Subsystem ==
  note: Reoptimzation Limit Sitting
  BattSOC_frac : Inport
  DP_OptSOCVec : Inport  Port=2
  Abs : Abs
  Assertion : Assertion  AssertionFailFcn=set_param(bdroot,'SimulationCommand','pause');  StopWhenAssertionFail=off
  Compare To Constant : simulink/Logic and Bit Operations/Compare To Constant  relop=>  const=0.03  OutDataTypeStr=boolean
  Constant3 : Constant
  Selector : Selector  InputPortWidth=30  IndexOptions=Index vector (port)  Indices=[1 3]  OutputSizes=1
  Subtract : Sum  Inputs=+-
  Terminator7 : Terminator
  To Workspace : ToWorkspace  VariableName=optSOCfrac  SaveFormat=Timeseries  SampleTime=-1
  Wait : Stateflow chart  TreatAsAtomicUnit=on
  wires:
  Selector/1 -> Subtract/2, To Workspace/1  "optSOCfrac"
  Constant3/1 -> Selector/2
  DP_OptSOCVec/1 -> Selector/1
  Wait/1(Trigger) -> Assertion/1  "ReOpt_Trigger"
  Subtract/1 -> Abs/1
  Abs/1 -> Compare To Constant/1
  Wait/2(Counter) -> Terminator7/1  "ctr"
  Compare To Constant/1 -> Wait/1(ReOptReq)  "ReOptimizeFlag"
  BattSOC_frac/1 -> Subtract/1

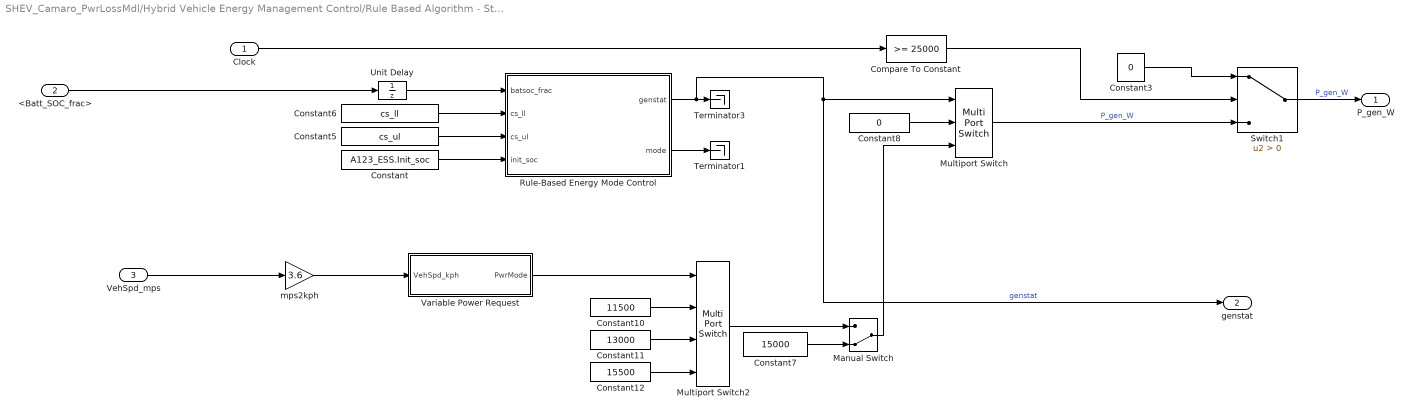
== system SHEV_Camaro_PwrLossMdl/Hybrid Vehicle Energy Management Control/Rule Based Algorithm - Standard ==
  Clock : Inport
  <Batt_SOC_frac> : Inport  Port=2
  VehSpd_mps : Inport  Port=3
  Compare To Constant : simulink/Logic and Bit Operations/Compare To Constant  relop=>=  const=25000  OutDataTypeStr=boolean
  Constant : Constant  Value=A123_ESS.Init_soc
  Constant10 : Constant  Value=11500
  Constant11 : Constant  Value=13000
  Constant12 : Constant  Value=15500
  Constant3 : Constant  Value=0
  Constant5 : Constant  Value=cs_ul
  Constant6 : Constant  Value=cs_ll
  Constant7 : Constant  Value=15000
  Constant8 : Constant  Value=0
  Manual Switch : ManualSwitch  CurrentSetting=0
  Multiport Switch : MultiPortSwitch  DataPortOrder=Zero-based contiguous  Inputs=2  zeroidx=on
  Multiport Switch2 : MultiPortSwitch  DataPortOrder=Zero-based contiguous  zeroidx=on
  Rule-Based Energy Mode Control : Stateflow chart  TreatAsAtomicUnit=on
  Switch1 : Switch  Criteria=u2 > Threshold
  Terminator1 : Terminator
  Terminator3 : Terminator
  Unit Delay : UnitDelay  SampleTime=-1
  Variable Power Request : MATLAB Function  TreatAsAtomicUnit=on
  mps2kph : Gain  Gain=3.6
  P_gen_W : Outport
  genstat : Outport  Port=2
  wires:
  Multiport Switch2/1 -> Manual Switch/1
  Constant12/1 -> Multiport Switch2/4
  Constant11/1 -> Multiport Switch2/3
  Variable Power Request/1(PwrMode) -> Multiport Switch2/1
  Constant3/1 -> Switch1/1
  <Batt_SOC_frac>/1 -> Unit Delay/1
  Constant/1 -> Rule-Based Energy Mode Control/4(init_soc)
  Constant10/1 -> Multiport Switch2/2
  Constant8/1 -> Multiport Switch/2
  Clock/1 -> Compare To Constant/1
  Rule-Based Energy Mode Control/2(mode) -> Terminator1/1
  Constant7/1 -> Manual Switch/2
  Rule-Based Energy Mode Control/1(genstat) -> genstat/1, Multiport Switch/1, Terminator3/1  "genstat"
  VehSpd_mps/1 -> mps2kph/1
  Unit Delay/1 -> Rule-Based Energy Mode Control/1(batsoc_frac)
  mps2kph/1 -> Variable Power Request/1(VehSpd_kph)
  Constant5/1 -> Rule-Based Energy Mode Control/3(cs_ul)
  Compare To Constant/1 -> Switch1/2
  Multiport Switch/1 -> Switch1/3  "P_gen_W"
  Constant6/1 -> Rule-Based Energy Mode Control/2(cs_ll)
  Manual Switch/1 -> Multiport Switch/3
  Switch1/1 -> P_gen_W/1  "P_gen_W"

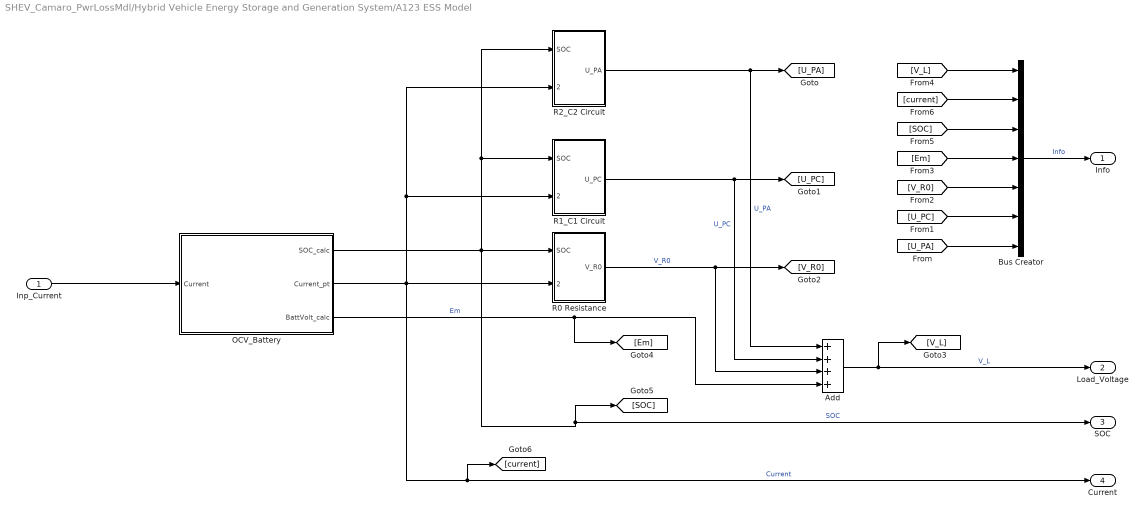
== system SHEV_Camaro_PwrLossMdl/Hybrid Vehicle Energy Storage and Generation System/A123 ESS Model ==
  Inp_Current : Inport
  Add : Sum  Inputs=++++
  Bus Creator : BusCreator  Inputs=7
  OCV_Battery : Subsystem
  R0 Resistance : Subsystem
  R1_C1 Circuit : Subsystem
  R2_C2 Circuit : Subsystem
  Info : Outport
  Load_Voltage : Outport  Port=2
  SOC : Outport  Port=3
  Current : Outport  Port=4
  wires:
  [SOC] -> Bus Creator/3
  [U_PA] -> Bus Creator/7
  Inp_Current/1 -> OCV_Battery/1(Current)
  [current] -> Bus Creator/2
  Add/1 -> Load_Voltage/1, [V_L]  "V_L"
  [Em] -> Bus Creator/4
  R0 Resistance/1(V_R0) -> [V_R0], Add/3  "V_R0"
  R2_C2 Circuit/1(U_PA) -> Add/1, [U_PA]  "U_PA"
  OCV_Battery/2(Current_pt) -> Current/1, [current], R2_C2 Circuit/2(Current), R1_C1 Circuit/2(Current), R0 Resistance/2(Current)  "Current"
  OCV_Battery/1(SOC_calc) -> SOC/1, [SOC], R2_C2 Circuit/1(SOC), R1_C1 Circuit/1(SOC), R0 Resistance/1(SOC)  "SOC"
  R1_C1 Circuit/1(U_PC) -> Add/2, [U_PC]  "U_PC"
  [U_PC] -> Bus Creator/6
  OCV_Battery/3(BattVolt_calc) -> [Em], Add/4  "Em"
  [V_R0] -> Bus Creator/5
  Bus Creator/1 -> Info/1  "Info"
  [V_L] -> Bus Creator/1

== system SHEV_Camaro_PwrLossMdl/Hybrid Vehicle Energy Storage and Generation System/Battery EPO Logic ==
  note: Discharge Current is negative
  Batt_SOC_frac : Inport
  LoadCurrent_A : Inport  Port=2
  10-second average : dspstat3/Moving Average  Method=Sliding window  ForgettingFactorPort=off  SpecifyWindowLength=on  WindowLength=1000  ForgettingFactor=0.9  SimulateUsing=Code generation
  10sec Discharge Limit Table A123 : Lookup_n-D  BreakpointsForDimension1=A123_ESS.cellTempbpt_C  BreakpointsForDimension2=A123_ESS.socbpt  Table=A123_ESS.DchgCurrLim_10sAvg_A  InternalRulePriority=Speed  RndMeth=Simplest  InputSameDT=on
  Battery EPO Constraint Logic : Stateflow chart  TreatAsAtomicUnit=on
  CellTemp degC : Constant  Value=35
  Gain1 : Gain  Gain=-1
  Batt_EPO : Outport
  wires:
  Batt_SOC_frac/1 -> 10sec Discharge Limit Table A123/2
  LoadCurrent_A/1 -> 10-second average/1
  Battery EPO Constraint Logic/1(epo_flag) -> Batt_EPO/1  "Batt_EPO"
  10-second average/1 -> Battery EPO Constraint Logic/2(LoadCurr)  "LoadCurrent_10sAvg_A"
  CellTemp degC/1 -> 10sec Discharge Limit Table A123/1
  Gain1/1 -> Battery EPO Constraint Logic/1(DchgCurrLim)
  10sec Discharge Limit Table A123/1 -> Gain1/1

== system SHEV_Camaro_PwrLossMdl/Hybrid Vehicle Energy Storage and Generation System/Fuel Level Calculator ==
  mfuel_gps : Inport
  Constant : Constant  Value=V_fuel_init_gal
  Discrete-Time Integrator : DiscreteIntegrator  SampleTime=-1  ICPrevOutput=DiscIntNeverNeededParam  ICPrevScaledInput=DiscIntNeverNeededParam
  Divide1 : Product  Inputs=*/
  Fuel Density : Gain  Gain=(0.2642/rho_fuel_gpL)
  Gain1 : Gain  Gain=100
  Subtract : Sum  Inputs=+-
  USGal2Liter : Gain  Gain=3.78541
  fuelLvl_pct : Outport
  fuelUsed_L : Outport  Port=2
  wires:
  Divide1/1 -> Gain1/1
  Subtract/1 -> Divide1/1  "fuelLeft_gal"
  Fuel Density/1 -> USGal2Liter/1, Subtract/2  "fuelUsed_gal"
  Constant/1 -> Divide1/2, Subtract/1
  Discrete-Time Integrator/1 -> Fuel Density/1  "mfuel_g"
  mfuel_gps/1 -> Discrete-Time Integrator/1
  Gain1/1 -> fuelLvl_pct/1  "fuelLvl_pct"
  USGal2Liter/1 -> fuelUsed_L/1  "fuelUsed_L"

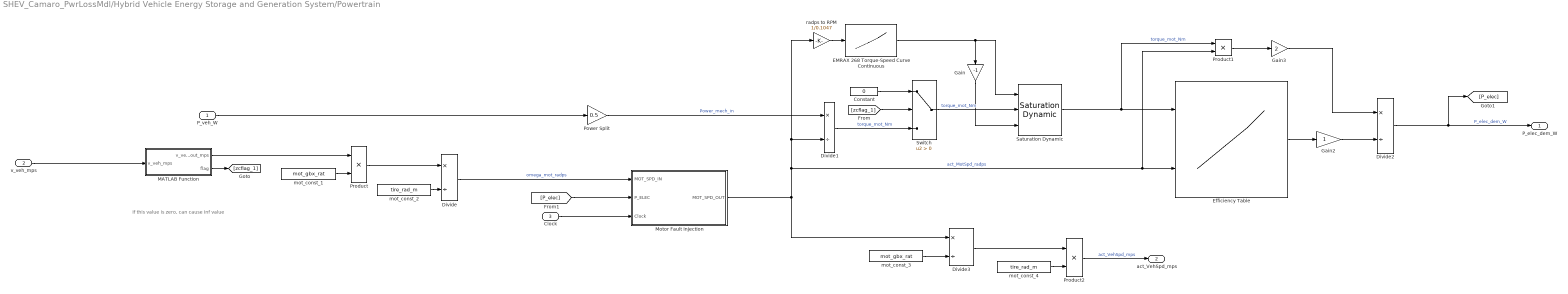
== system SHEV_Camaro_PwrLossMdl/Hybrid Vehicle Energy Storage and Generation System/Powertrain ==
  note: If this value is zero, can cause Inf value
  P_veh_W : Inport
  v_veh_mps : Inport  Port=2
  Clock : Inport  Port=3
  Constant : Constant  Value=0
  Divide{,1..3} (4 alike) : Product  Inputs=*/
  EMRAX 268 Torque-Speed Curve Continuous : Lookup_n-D  NumberOfTableDimensions=1  BreakpointsForDimension1=motSpdVec  Table=contMotTrq  InternalRulePriority=Speed  RndMeth=Simplest  InputSameDT=on
  Efficiency Table : Lookup_n-D  BreakpointsForDimension1=motTrqVec  BreakpointsForDimension2=motSpdVec  Table=adj_motEffMap  ExtrapMethod=Clip  UseLastTableValue=on  InternalRulePriority=Speed  RndMeth=Simplest  InputSameDT=on
  Gain : Gain  Gain=-1
  Gain2 : Gain
  Gain3 : Gain  Gain=2
  MATLAB Function : MATLAB Function  TreatAsAtomicUnit=on
  Motor Fault Injection : Subsystem  mask{FaultDec=off, P_derate=30000, t_fault=6000, contMotTrqMax=180}
      mask prompts: FaultDec "Select to enable motor deration fault."; P_derate "Enter the motor deration power [Watts]:"; t_fault "Time for fault insertion [seconds]:"; contMotTrqMax "Maximum Continuous Motor Torque [Nm]:"
      mask DialogControl DescGroupVar Prompt: Motor Fault Injection
      mask DialogControl DescTextVar Prompt: Use the parameter controls to induce a deration fault in the motor subsystem.
  Power Split : Gain  Gain=0.5
  Product : Product
  Product1 : Product
  Product2 : Product
  Saturation Dynamic : simulink/Discontinuities/Saturation Dynamic  OutMin=[]  OutMax=[]  OutDataTypeStr=Inherit: Same as second input  OutDataType=fixdt(1, 16)  OutScaling=2^-10  DoSatur=off
  Switch : Switch  Criteria=u2 > Threshold
  mot_const_1 : Constant  Value=mot_gbx_rat
  mot_const_2 : Constant  Value=tire_rad_m
  mot_const_3 : Constant  Value=mot_gbx_rat
  mot_const_4 : Constant  Value=tire_rad_m
  radps to RPM : Gain  Gain=1/0.1047
  P_elec_dem_W : Outport
  act_VehSpd_mps : Outport  Port=2
  wires:
  Saturation Dynamic/1 -> Product1/1, Efficiency Table/1  "torque_mot_Nm"
  [zcflag_1] -> Switch/2
  Product/1 -> Divide/1
  radps to RPM/1 -> EMRAX 268 Torque-Speed Curve Continuous/1
  Constant/1 -> Switch/1
  MATLAB Function/1(v_veh_out_mps) -> Product/1
  Gain/1 -> Saturation Dynamic/3
  mot_const_1/1 -> Product/2
  EMRAX 268 Torque-Speed Curve Continuous/1 -> Gain/1, Saturation Dynamic/1
  Power Split/1 -> Divide1/1  "Power_mech_in"
  v_veh_mps/1 -> MATLAB Function/1(v_veh_mps)
  P_veh_W/1 -> Power Split/1
  Efficiency Table/1 -> Gain2/1
  Switch/1 -> Saturation Dynamic/2  "torque_mot_Nm"
  mot_const_2/1 -> Divide/2
  MATLAB Function/2(flag) -> [zcflag_1]
  Product1/1 -> Gain3/1
  Divide2/1 -> [P_elec], P_elec_dem_W/1  "P_elec_dem_W"
  Gain2/1 -> Divide2/2
  Gain3/1 -> Divide2/1
  Divide1/1 -> Switch/3  "torque_mot_Nm"
  Motor Fault Injection/1(MOT_SPD_OUT) -> Product1/2, Efficiency Table/2, Divide1/2, radps to RPM/1, Divide3/1  "act_MotSpd_radps"
  Divide/1 -> Motor Fault Injection/1(MOT_SPD_IN)  "omega_mot_radps"
  [P_elec] -> Motor Fault Injection/2(P_ELEC)
  Clock/1 -> Motor Fault Injection/3(Clock)
  mot_const_3/1 -> Divide3/2
  Divide3/1 -> Product2/1
  mot_const_4/1 -> Product2/2
  Product2/1 -> act_VehSpd_mps/1  "act_VehSpd_mps"

== system SHEV_Camaro_PwrLossMdl/Hybrid Vehicle Energy Storage and Generation System/A123 ESS Model/OCV_Battery ==
  note: Intial SOC value goes in this memory block
  Current : Inport
  Add : Sum
  Constant : Constant  Value=Ns
  Constant1 : Constant  Value=Q_max_cell * Np
  Constant2 : Constant  Value=Nmod
  Divide : Product  Inputs=*/
  Gain : Gain  Gain=t_step/3600
  Memory : Memory  InitialCondition=soc_init  InheritSampleTime=on  LinearizeAsDelay=on
  OCV Function : MATLAB Function  TreatAsAtomicUnit=on
  Product : Product  Inputs=3
  SOC_calc : Outport
  Current_pt : Outport  Port=2
  BattVolt_calc : Outport  Port=3
  wires:
  Current/1 -> OCV Function/2(current), Current_pt/1, Gain/1
  Gain/1 -> Divide/1
  Memory/1 -> Add/1
  Constant2/1 -> Product/3
  OCV Function/1(ocv) -> Product/1  "OCV_calc"
  Constant1/1 -> Divide/2
  Add/1 -> SOC_calc/1, OCV Function/1(soc), Memory/1  "SOC_calc"
  Constant/1 -> Product/2
  Divide/1 -> Add/2
  Product/1 -> BattVolt_calc/1  "BattVolt_calc"

== system SHEV_Camaro_PwrLossMdl/Hybrid Vehicle Energy Storage and Generation System/A123 ESS Model/R0 Resistance ==
  SOC : Inport
  Current : Inport  Port=2
  Compare To Zero : simulink/Logic and Bit Operations/Compare To Zero  relop=>  OutDataTypeStr=boolean
  Product : Product
  R0 LUT Chg : Lookup_n-D  NumberOfTableDimensions=1  BreakpointsForDimension1=soc_bpt  Table=R0 * 0.05  InternalRulePriority=Speed  RndMeth=Simplest  InputSameDT=on
  R0 LUT Dchg : Lookup_n-D  NumberOfTableDimensions=1  BreakpointsForDimension1=soc_bpt  Table=R0*0.25  InternalRulePriority=Speed  RndMeth=Simplest  InputSameDT=on
  Switch : Switch  Criteria=u2 > Threshold
  V_R0 : Outport
  wires:
  R0 LUT Chg/1 -> Switch/1  "R0"
  SOC/1 -> R0 LUT Chg/1, R0 LUT Dchg/1
  Current/1 -> Compare To Zero/1, Product/2
  Product/1 -> V_R0/1
  Switch/1 -> Product/1
  Compare To Zero/1 -> Switch/2
  R0 LUT Dchg/1 -> Switch/3  "R0"

== system SHEV_Camaro_PwrLossMdl/Hybrid Vehicle Energy Storage and Generation System/A123 ESS Model/R1_C1 Circuit ==
  SOC : Inport
  Current : Inport  Port=2
  Add1 : Sum
  C1 LUT : Lookup_n-D  NumberOfTableDimensions=1  BreakpointsForDimension1=soc_bpt  Table=C1  InternalRulePriority=Speed  RndMeth=Simplest  InputSameDT=on
  Discrete-Time Integrator : DiscreteIntegrator  SampleTime=-1  ICPrevOutput=DiscIntNeverNeededParam  ICPrevScaledInput=DiscIntNeverNeededParam
  Divide : Product  Inputs=*/
  Divide1 : Product  Inputs=*/
  Product : Product
  R1 LUT : Lookup_n-D  NumberOfTableDimensions=1  BreakpointsForDimension1=soc_bpt  Table=R1  InternalRulePriority=Speed  RndMeth=Simplest  InputSameDT=on
  U_PC : Outport
  wires:
  Product/1 -> Divide1/2
  SOC/1 -> R1 LUT/1, C1 LUT/1
  Divide1/1 -> Add1/1
  C1 LUT/1 -> Product/2, Divide/2
  Divide/1 -> Add1/2
  R1 LUT/1 -> Product/1
  Discrete-Time Integrator/1 -> U_PC/1, Divide1/1  "U_PC"
  Add1/1 -> Discrete-Time Integrator/1  "U_PC_derivative"
  Current/1 -> Divide/1

== system SHEV_Camaro_PwrLossMdl/Hybrid Vehicle Energy Storage and Generation System/A123 ESS Model/R2_C2 Circuit ==
  SOC : Inport
  Current : Inport  Port=2
  Add1 : Sum
  C2 LUT : Lookup_n-D  NumberOfTableDimensions=1  BreakpointsForDimension1=soc_bpt  Table=C2  InternalRulePriority=Speed  RndMeth=Simplest  InputSameDT=on
  Discrete-Time Integrator : DiscreteIntegrator  SampleTime=-1  ICPrevOutput=DiscIntNeverNeededParam  ICPrevScaledInput=DiscIntNeverNeededParam
  Divide : Product  Inputs=*/
  Divide1 : Product  Inputs=*/
  Product : Product
  R2 LUT : Lookup_n-D  NumberOfTableDimensions=1  BreakpointsForDimension1=soc_bpt  Table=R2  InternalRulePriority=Speed  RndMeth=Simplest  InputSameDT=on
  U_PA : Outport
  wires:
  Product/1 -> Divide1/2
  SOC/1 -> R2 LUT/1, C2 LUT/1
  Divide1/1 -> Add1/1
  C2 LUT/1 -> Product/2, Divide/2
  Divide/1 -> Add1/2
  R2 LUT/1 -> Product/1
  Discrete-Time Integrator/1 -> U_PA/1, Divide1/1  "U_PA"
  Add1/1 -> Discrete-Time Integrator/1  "U_PA_derivative"
  Current/1 -> Divide/1
